simulink model "motor"  (R2026a)
settings: Solver=VariableStepAuto
undefined symbols (not defined in the file): pmsm
libraries: autolibpmsminterior x1
settings Model: Creator=probst  LastModifiedBy=probst

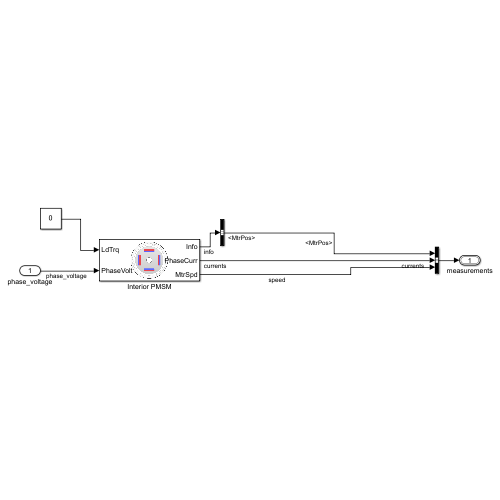
[thumbnail: Simulink's stored preview of the top-level diagram]
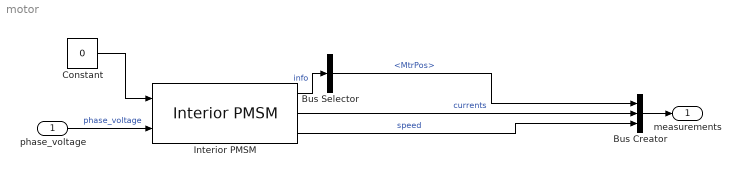
== system motor ==
  phase_voltage : Inport
  Bus Creator : BusCreator  Inputs=3  OutDataTypeStr=Bus: plant_measurement  NonVirtualBus=on
  Bus Selector : BusSelector  OutputSignals=MtrPos
  Constant : Constant  Value=0
  Interior PMSM : autolibpmsminterior/Interior PMSM  port_config=Torque  sim_type=Continuous  Ts=0.001  P=pmsm.P  Rs=pmsm.Rs  Ldq=pmsm.Ldq  KConstText=Permanent flux linkage constant (lambda_pm):  lambda_pm=pmsm.fl  Ke=pmsm.Ke  mechanical=pmsm.mechanical  idq0=[0 0]  theta_init=0  omega_init=0  KConst=pmsm.fl  lambda_pm_calc=pmsm.fl  Kt=0.07  RefBlkName='autolibpmsminterior/Interior PMSM'  aMode=5
      settings: LibrarySourceBlock=mcblib/Electrical Systems/Motors/Interior PMSM
  measurements : Outport  OutDataTypeStr=Bus: plant_measurement
  wires:
  Bus Selector/1 -> Bus Creator/1  "<MtrPos>"
  Bus Creator/1 -> measurements/1
  Interior PMSM/1 -> Bus Selector/1  "info"
  Interior PMSM/3 -> Bus Creator/3  "speed"
  Constant/1 -> Interior PMSM/1
  Interior PMSM/2 -> Bus Creator/2  "currents"
  phase_voltage/1 -> Interior PMSM/2  "phase_voltage"
